simulink model "Lab6S"  (R2018a)
settings: Solver=VariableStepAuto  StartTime=0.0  StopTime=50.0  MaxStep=0.005  RelTol=1e-3
values from neighbouring files (symbols this model uses):
  A1 = k(1)    [Lab6.m]    (also in script7.m = 1; test.m)
  a1 = Aw1 * sqrt( 2 * g * H1max ) / H1max    [Lab6.m]
  A2 = k(1)    [Lab6.m]    (also in script7.m = 1; test.m)
  a2 = Aw2 * sqrt( 2 * g * H2max ) / H2max    [Lab6.m]
  delay = 10    [Lab6.m]
  Fw1 = FWe10(i)    [Lab6.m]
  FW1max = Aw1 * sqrt( 2 * g * ( H1max - H2max ) )    [Lab6.m]
  Fw2 = FWe20(i)    [Lab6.m]
  FW2max = Aw2 * sqrt( 2 * g * H2max ) - 0    [Lab6.m]
  H10 = Fw1^2/(2*Aw1^2*g) + H20    [Lab6.m]
  H20 = ((Fw1 + Fw2)^2) / (2*(Aw2^2)*g)    [Lab6.m]
settings Model: Creator=aplov  LastModifiedBy=aplov

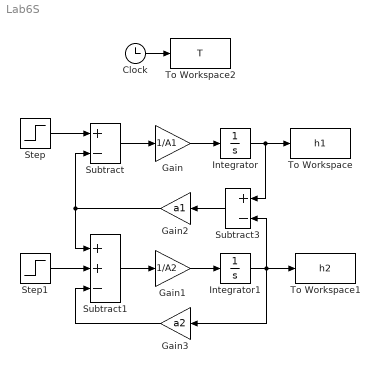
== system Lab6S ==
  Clock : Clock
  Gain : Gain  Gain=1/A1
  Gain1 : Gain  Gain=1/A2
  Gain2 : Gain  Gain=a1
  Gain3 : Gain  Gain=a2
  Integrator : Integrator  InitialCondition=H10
  Integrator1 : Integrator  InitialCondition=H20
  Step : Step  Time=delay  Before=Fw1  After=Fw1 + 0.1*FW1max  SampleTime=0
  Step1 : Step  Time=delay  Before=Fw2  After=Fw2 + FW2max  SampleTime=0
  Subtract : Sum  Inputs=+-
  Subtract1 : Sum  Inputs=++-
  Subtract3 : Sum  Inputs=+-
  To Workspace : ToWorkspace  VariableName=h1  SampleTime=-1
  To Workspace1 : ToWorkspace  VariableName=h2  SampleTime=-1
  To Workspace2 : ToWorkspace  VariableName=T  SampleTime=-1
  wires:
  Step/1 -> Subtract/1
  Subtract/1 -> Gain/1
  Gain/1 -> Integrator/1
  Integrator/1 -> Subtract3/1, To Workspace/1
  Subtract1/1 -> Gain1/1
  Gain1/1 -> Integrator1/1
  Subtract3/1 -> Gain2/1
  Integrator1/1 -> Gain3/1, Subtract3/2, To Workspace1/1
  Step1/1 -> Subtract1/2
  Gain2/1 -> Subtract1/1, Subtract/2
  Gain3/1 -> Subtract1/3
  Clock/1 -> To Workspace2/1
